simulink model "double_pendulum"  (R2020b)
settings: Solver=ode113  StartTime=0.0  StopTime=180  FixedStep=0.001  MaxStep=0.01  RelTol=1e-3
InitFcn:
  | q1 = 0;
  | q2 = 0;
  | omega1 = 0;
  | omega2 = 0;
settings Model: Creator=stardust  LastModifiedBy=stardust

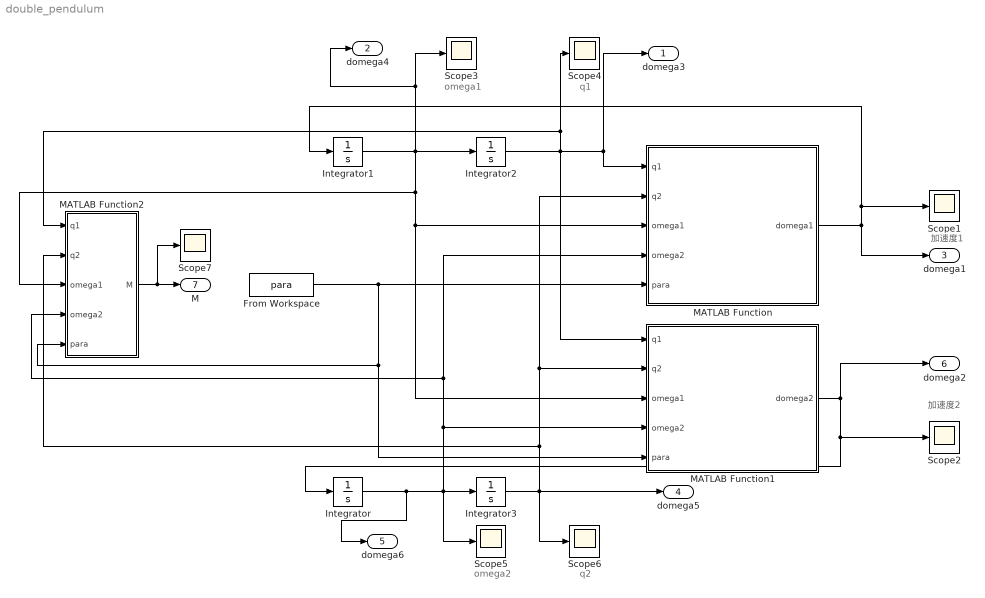
== system double_pendulum ==
  note: 加速度2
  note: 加速度1
  note: omega1
  note: omega2
  note: q2
  note: q1
  From Workspace : FromWorkspace  VariableName=para
  Integrator{,1..3} (4 alike) : Integrator
  MATLAB Function : MATLAB Function  TreatAsAtomicUnit=on
  MATLAB Function1 : MATLAB Function  TreatAsAtomicUnit=on
  MATLAB Function2 : MATLAB Function  TreatAsAtomicUnit=on
  Scope{1..7} (7 alike) : Scope
  domega3 : Outport  SignalName=q1
  domega4 : Outport  Port=2  SignalName=omega1
  domega1 : Outport  Port=3  SignalName=domega1
  domega5 : Outport  Port=4  SignalName=q2
  domega6 : Outport  Port=5  SignalName=omega2
  domega2 : Outport  Port=6  SignalName=domega2
  M : Outport  Port=7  SignalName=M
  wires:
  MATLAB Function/1(domega1) -> Integrator1/1, Scope1/1, domega1/1
  MATLAB Function1/1(domega2) -> domega2/1, Scope2/1, Integrator/1
  Integrator2/1 -> MATLAB Function2/1(q1), Scope4/1, MATLAB Function1/1(q1), domega3/1, MATLAB Function/1(q1)
  Integrator/1 -> domega6/1, Scope5/1, MATLAB Function/4(omega2), MATLAB Function2/4(omega2), MATLAB Function1/4(omega2), Integrator3/1
  Integrator3/1 -> Scope6/1, domega5/1, MATLAB Function2/2(q2), MATLAB Function/2(q2), MATLAB Function1/2(q2)
  Integrator1/1 -> domega4/1, Scope3/1, MATLAB Function2/3(omega1), MATLAB Function1/3(omega1), MATLAB Function/3(omega1), Integrator2/1
  From Workspace/1 -> MATLAB Function2/5(para), MATLAB Function1/5(para), MATLAB Function/5(para)
  MATLAB Function2/1(M) -> Scope7/1, M/1

== matlab function double_pendulum/MATLAB Function1 ==
  data: q1 input; domega2 output; q2 input; omega1 input; omega2 input; para input
function domega2 = fcn(q1,q2, omega1, omega2,para)
% l1 = 0.05; l2 = 0.025; c = 0.05; % 要优化的参数
l1 = para(1); l2 = para(2); c = para(3);
t1 = 0.15/2-l1; t2 = 0.1/2 - l2; m1 = 0.6; m2 = 0.5; 
J1 = 0.001125;J2 = 0.0004167; g = 9.8;
A = m1*t1^2+m2*l1^2+J1;
B = -m2*t2*l1*cos(q1-q2);
C = (m1*t1-m2*l1)*g*cos(q1)+c*omega1-m2*t2*l1*sin(q1-q2)*omega2^2;
E = m2*t2^2+J2;
D = -m2*t2*l1*cos(q1-q2);
F = m2*t2*l1*sin(q1-q2)*omega1^2+m2*t2*g*cos(q2)+c*omega2;
domega2 = (A*F-C*D)*E/(D*B-E*A);

== matlab function double_pendulum/MATLAB Function ==
  data: q1 input; domega1 output; q2 input; omega1 input; omega2 input; para input
function domega1 = fcn(q1,q2, omega1, omega2,para)
% l1 = 0.05; l2 = 0.025; c = 0.05; % 要优化的参数
l1 = para(1); l2 = para(2); c = para(3);
t1 = 0.15/2-l1; t2 = 0.1/2 - l2; m1 = 0.6; m2 = 0.5; 
J1 = 0.001125;J2 = 0.0004167; g = 9.8;
A = m1*t1^2+m2*l1^2+J1;
B = -m2*t2*l1*cos(q1-q2);
C = (m1*t1-m2*l1)*g*cos(q1)+c*omega1-m2*t2*l1*sin(q1-q2)*omega2^2;
E = m2*t2^2+J2;
D = -m2*t2*l1*cos(q1-q2);
F = m2*t2*l1*sin(q1-q2)*omega1^2+m2*t2*g*cos(q2)+c*omega2;
domega1 = (C*E-F*B)/(D*B-E*A);

== matlab function double_pendulum/MATLAB Function2 ==
  data: q1 input; M output; q2 input; omega1 input; omega2 input; para input
function M = fcn(q1,q2, omega1, omega2,para)
l1 = para(1); l2 = para(2);
lDE = 0.15; lGF = 0.1;
t1 = lDE/2-l1; t2 = lGF/2 - l2; m1 = 0.6; m2 = 0.5; 
J1 = 0.001125;J2 = 0.0004167; g = 9.8;
y1 = t1*sin(q1); y2 = -l1*sin(q1)+t2*sin(q2);
M = m1*t1^2*omega1^2/2 + m2/2*(l1^2*omega1^2+t2^2*omega2^2-2*t2*l1*omega1*omega2*cos(q1-q2))+ J1*omega1^2/2 + J2*omega2^2/2 + m1*g*(y1+5) + m2*g*(y2+5);
